simulink model "quadcopter_PD"  (R2015b)
settings: Solver=VariableStepAuto  StartTime=0.0  StopTime=2.0  MaxStep=1e-2  RelTol=1e-3
undefined symbols (not defined in the file): A, b, g, I, Im, k, Kphi, Kpsi, Ktheta, Kz, l, m, Tdphi, Tdpsi, Tdtheta, Tdz
libraries: simulink x2
settings Model: Creator=mgreiff  LastModifiedBy=mgreiff

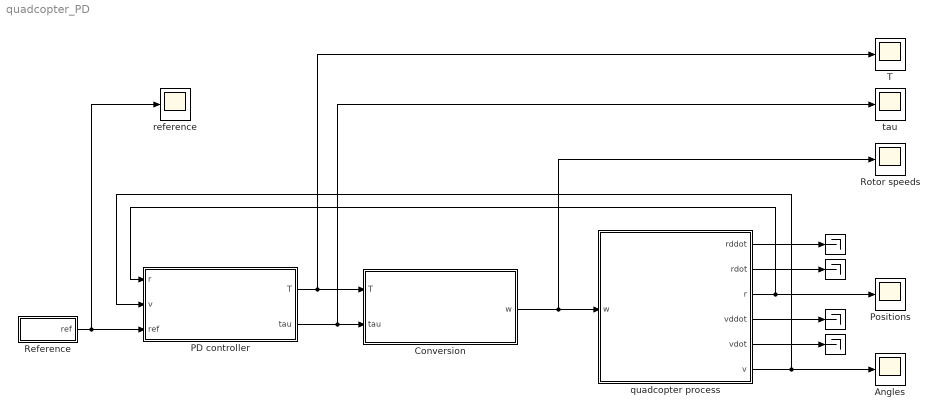
== system quadcopter_PD ==
  " " : Terminator
  "  " : Terminator
  "   " : Terminator
  "     " : Terminator
  Angles : Scope
  Conversion : Subsystem
  PD controller : Subsystem
  Positions : Scope
  Reference : Subsystem
  Rotor speeds : Scope
  T : Scope
  quadcopter process : Subsystem
  reference : Scope
  tau : Scope
  wires:
  quadcopter process/3(r) -> PD controller/1(r), Positions/1
  quadcopter process/6(v) -> PD controller/2(v), Angles/1
  Conversion/1(w) -> quadcopter process/1(w), Rotor speeds/1
  quadcopter process/5(vdot) -> "  "/1
  quadcopter process/4(vddot) -> " "/1
  quadcopter process/2(rdot) -> "   "/1
  quadcopter process/1(rddot) -> "     "/1
  PD controller/1(T) -> T/1, Conversion/1(T)
  PD controller/2(tau) -> tau/1, Conversion/2(tau)
  Reference/1(ref) -> reference/1, PD controller/3(ref)

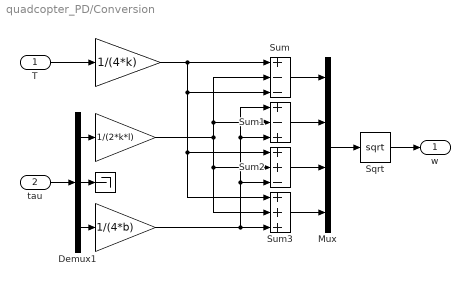
== system quadcopter_PD/Conversion ==
  T : Inport
  tau : Inport  Port=2
  " " : Terminator
  "  " : Gain  Gain=1/(4*k)
  "    " : Gain  Gain=1/(2*k*l)
  "       " : Gain  Gain=1/(4*b)
  Demux1 : Demux  Outputs=3
  Mux : Mux
  Sqrt : Sqrt  SaturateOnIntegerOverflow=on
  Sum : Sum  Inputs=+--
  Sum1 : Sum  Inputs=+-+
  Sum2 : Sum  Inputs=++-
  Sum3 : Sum  Inputs=+++
  w : Outport
  wires:
  tau/1 -> Demux1/1
  Demux1/2 -> " "/1
  T/1 -> "  "/1
  Demux1/1 -> "    "/1
  Demux1/3 -> "       "/1
  Mux/1 -> Sqrt/1
  Sum/1 -> Mux/1
  "  "/1 -> Sum3/1, Sum2/1, Sum/3, Sum/1
  Sum1/1 -> Mux/2
  Sum2/1 -> Mux/3
  Sum3/1 -> Mux/4
  "       "/1 -> Sum1/1, Sum1/3, Sum2/3, Sum3/3
  "    "/1 -> Sum/2, Sum1/2, Sum3/2, Sum2/2
  Sqrt/1 -> w/1

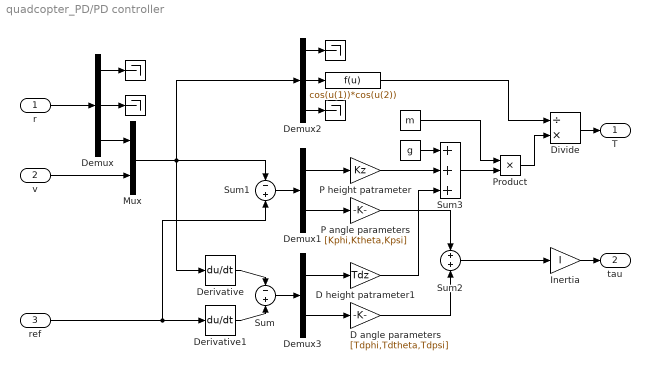
== system quadcopter_PD/PD controller ==
  r : Inport
  v : Inport  Port=2
  ref : Inport  Port=3
  " " : Terminator
  "  " : Terminator
  "    " : Terminator
  "     " : Constant  Value=m
  "      " : Constant  Value=g
  "       " : Fcn  Expr=cos(u(1))*cos(u(2))
  "            " : Terminator
  D angle parameters : Gain  Gain=[Tdphi,Tdtheta,Tdpsi]
  D height patrameter1 : Gain  Gain=Tdz
  Demux : Demux  Outputs=3
  Demux1 : Demux  Outputs=[1,3]
  Demux2 : Demux  Outputs=[1,2,1]
  Demux3 : Demux  Outputs=[1,3]
  Derivative : Derivative
  Derivative1 : Derivative
  Divide : Product  Inputs=/*
  Inertia : Gain  Gain=I
  Mux : Mux  Inputs=2
  P angle parameters : Gain  Gain=[Kphi,Ktheta,Kpsi]
  P height patrameter : Gain  Gain=Kz
  Product : Product
  Sum : Sum  Inputs=-+
  Sum1 : Sum  Inputs=-+
  Sum2 : Sum
  Sum3 : Sum  Inputs=+++
  T : Outport
  tau : Outport  Port=2
  wires:
  Demux/1 -> "  "/1
  Demux/2 -> " "/1
  r/1 -> Demux/1
  Demux/3 -> Mux/1
  v/1 -> Mux/2
  Mux/1 -> Sum1/1, Demux2/1, Derivative/1
  ref/1 -> Sum1/2, Derivative1/1
  Derivative/1 -> Sum/1
  Derivative1/1 -> Sum/2
  Sum1/1 -> Demux1/1
  Sum/1 -> Demux3/1
  Demux1/2 -> P angle parameters/1
  Demux3/2 -> D angle parameters/1
  P angle parameters/1 -> Sum2/1
  D angle parameters/1 -> Sum2/2
  Sum2/1 -> Inertia/1
  Demux3/1 -> D height patrameter1/1
  Demux1/1 -> P height patrameter/1
  P height patrameter/1 -> Sum3/2
  D height patrameter1/1 -> Sum3/3
  "      "/1 -> Sum3/1
  Demux2/1 -> "    "/1
  Demux2/3 -> "            "/1
  Sum3/1 -> Product/2
  Demux2/2 -> "       "/1
  "     "/1 -> Product/1
  "       "/1 -> Divide/1
  Product/1 -> Divide/2
  Divide/1 -> T/1
  Inertia/1 -> tau/1

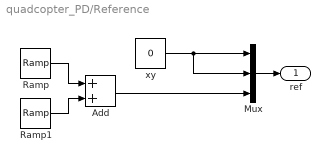
== system quadcopter_PD/Reference ==
  Add : Sum
  Mux : Mux  Inputs=3
  Ramp : simulink/Sources/Ramp  slope=1  start=0  X0=0
  Ramp1 : simulink/Sources/Ramp  slope=-1  start=1  X0=0
  xy : Constant  Value=0
  ref : Outport
  wires:
  Mux/1 -> ref/1
  xy/1 -> Mux/2, Mux/1
  Ramp/1 -> Add/1
  Add/1 -> Mux/3
  Ramp1/1 -> Add/2

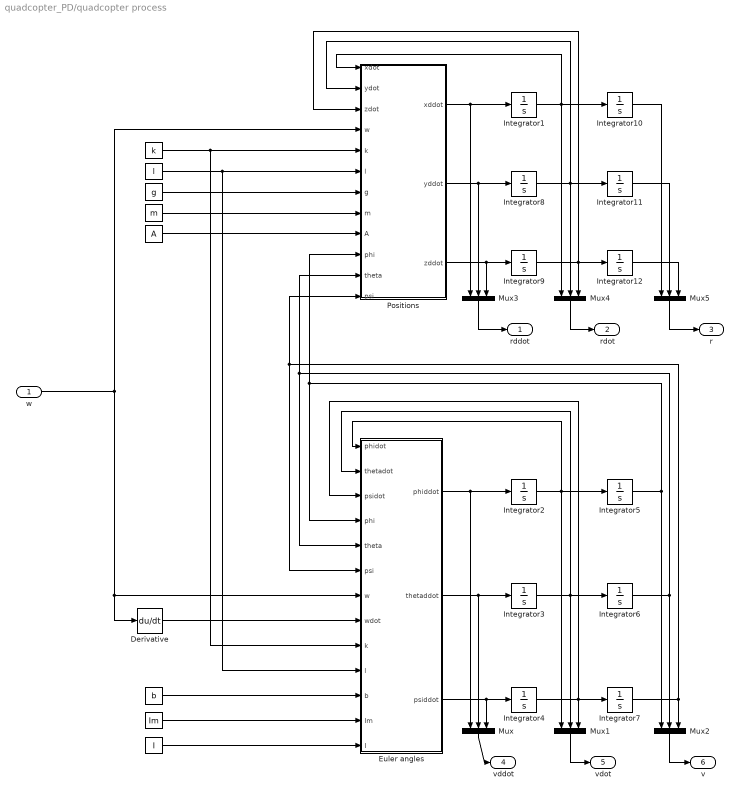
== system quadcopter_PD/quadcopter process ==
  w : Inport
  " " : Constant  Value=k
  "   " : Constant  Value=l
  "    " : Constant  Value=g
  "     " : Constant  Value=m
  "       " : Constant  Value=A
  "         " : Constant  Value=b
  "          " : Constant  Value=I
  "           " : Constant  Value=Im
  Derivative : Derivative
  Euler angles : MATLAB Function  TreatAsAtomicUnit=on
  Integrator{1..12} (12 alike) : Integrator
  Mux{,1..5} (6 alike) : Mux  Inputs=3
  Positions : MATLAB Function  TreatAsAtomicUnit=on
  rddot : Outport
  rdot : Outport  Port=2
  r : Outport  Port=3
  vddot : Outport  Port=4
  vdot : Outport  Port=5
  v : Outport  Port=6
  wires:
  " "/1 -> Positions/5(k), Euler angles/9(k)
  "    "/1 -> Positions/7(g)
  "   "/1 -> Positions/6(l), Euler angles/10(l)
  "     "/1 -> Positions/8(m)
  "       "/1 -> Positions/9(A)
  "         "/1 -> Euler angles/11(b)
  "          "/1 -> Euler angles/13(I)
  "           "/1 -> Euler angles/12(Im)
  Euler angles/1(phiddot) -> Mux/1, Integrator2/1
  Euler angles/2(thetaddot) -> Mux/2, Integrator3/1
  Euler angles/3(psiddot) -> Mux/3, Integrator4/1
  Mux/1 -> vddot/1
  Integrator4/1 -> Euler angles/3(psidot), Mux1/3, Integrator7/1
  Integrator3/1 -> Euler angles/2(thetadot), Integrator6/1, Mux1/2
  Integrator2/1 -> Mux1/1, Euler angles/1(phidot), Integrator5/1
  Mux1/1 -> vdot/1
  Mux2/1 -> v/1
  Integrator7/1 -> Mux2/3, Euler angles/6(psi), Positions/12(psi)
  Integrator6/1 -> Mux2/2, Positions/11(theta), Euler angles/5(theta)
  Integrator5/1 -> Mux2/1, Euler angles/4(phi), Positions/10(phi)
  Derivative/1 -> Euler angles/8(wdot)
  w/1 -> Positions/4(w), Euler angles/7(w), Derivative/1
  Positions/1(xddot) -> Mux3/1, Integrator1/1
  Positions/2(yddot) -> Mux3/2, Integrator8/1
  Positions/3(zddot) -> Mux3/3, Integrator9/1
  Mux3/1 -> rddot/1
  Integrator9/1 -> Positions/3(zdot), Mux4/3, Integrator12/1
  Integrator8/1 -> Positions/2(ydot), Integrator11/1, Mux4/2
  Integrator1/1 -> Positions/1(xdot), Mux4/1, Integrator10/1
  Mux4/1 -> rdot/1
  Mux5/1 -> r/1
  Integrator12/1 -> Mux5/3
  Integrator11/1 -> Mux5/2
  Integrator10/1 -> Mux5/1

== matlab function quadcopter_PD/quadcopter process/Euler angles ==
  data: phidot input; thetadot input; psidot input; phi input; theta input; psi input; w input; wdot input; phiddot output; k input; l input; thetaddot output; psiddot output; b input; Im input; I input
function [phiddot,thetaddot,psiddot] = fcn(phidot, thetadot, psidot, phi, theta, psi, w, wdot, k, l, b, Im, I)
%#codegen

vdot = [phidot;
        thetadot;
        psidot];

Ixx = I(1);
Iyy = I(2);
Izz = I(3);

taum = b*sum(w) + Im*sum(wdot); % Should be w^2?
taub = [l*k*(-w(2)^2 + w(4)^2);l*k*(-w(1)^2 + w(3)^2);taum];

% Declare J matrix
J = zeros(3);
J(1,1) = Ixx;
J(1,3) = -Ixx*sin(theta);
J(2,2) = Iyy*cos(phi).^2+Izz*sin(phi).^2;
J(2,3) = (Iyy-Izz)*cos(phi)*sin(phi)*cos(theta);
J(3,1) = -Ixx*sin(theta);
J(3,2) = (Iyy-Izz)*cos(phi)*sin(phi)*cos(theta);
J(3,3) = Ixx*sin(theta).^2+...
         Iyy*sin(phi).^2*cos(theta).^2+...
         Izz*cos(phi).^2*cos(theta).^2;

% Declare C-matrix
C = zeros(3);
C(1,2) = (Iyy-Izz)*(thetadot*cos(phi)*sin(phi)+psidot*sin(phi).^2*cos(theta))+...
         (Izz-Iyy)*(psidot*cos(phi).^2*cos(theta))+...
         -Ixx*psidot*cos(theta);

C(1,3) = (Izz-Iyy)*psidot*cos(phi)*sin(phi)*cos(theta).^2;

C(2,1) = (Izz-Iyy)*(thetadot*cos(phi)*sin(phi)+psidot*sin(phi)*cos(theta))+...
         (Iyy-Ixx)*(psidot*cos(phi).^2*cos(theta))+...
         Ixx*psidot*cos(theta);

C(2,2) = (Izz-Iyy)*phidot*cos(phi)*sin(phi);

C(2,3) = -Ixx*psidot*sin(theta)*cos(theta)+...
         Iyy*psidot*sin(phi).^2*sin(theta)*cos(theta)+...
         Izz*psidot*cos(phi).^2*sin(theta)*cos(theta);

C(3,1) = (Iyy-Izz)*psidot*cos(theta).^2*sin(phi)*cos(phi)+...
         -Ixx*thetadot*cos(theta);

C(3,2) = (Izz-Iyy)*(thetadot*cos(phi)*sin(phi)*sin(theta)+phidot*sin(phi).^2*cos(theta))+...
         (Iyy-Izz)*phidot*cos(phi).^2*cos(theta)+...
         Ixx*psidot*sin(theta)*cos(theta)+...
         -Iyy*psidot*sin(phi).^2*sin(theta)*cos(theta)+...
         -Izz*psidot*cos(phi).^2*sin(theta)*cos(theta);

C(3,3) = (Iyy-Izz)*phidot*cos(phi)*sin(phi)*cos(theta).^2+...
         -Iyy*thetadot*sin(phi).^2*cos(theta)*sin(theta)+...
         -Izz*thetadot*cos(phi).^2*cos(theta)*sin(theta)+...
         Ixx*thetadot*cos(theta)*sin(theta);
vddot = inv(J)*(taub - C*vdot);
phiddot = vddot(1);
thetaddot = vddot(2);
psiddot = vddot(3);

== matlab function quadcopter_PD/quadcopter process/Positions ==
  data: xdot input; ydot input; zdot input; w input; k input; l input; g input; m input; A input; xddot output; phi input; theta input; psi input; yddot output; zddot output
function [xddot, yddot, zddot] = fcn(xdot, ydot, zdot, w, k, l, g, m, A, phi, theta, psi)
%#codegen
rdot = [xdot;ydot;zdot];
T = k*l*sum(w.^2);
map = [cos(psi)*sin(theta)*cos(phi) + sin(psi)*sin(phi);
       sin(psi)*sin(theta)*cos(phi) - cos(psi)*sin(phi);
       cos(theta)*cos(phi)];
gf = -g*[0;0;1];
rddot = gf + T*map./m  - A.*rdot./m;
xddot = rddot(1);
yddot = rddot(2);
zddot = rddot(3);
